simulink model "AOCS_FDIR"  (R2020b)
settings: Solver=ode45  StartTime=0.0  StopTime=200  FixedStep=1e-4  MaxStep=0.25  RelTol=1e-8  AbsTol=1e-8
values from neighbouring files (symbols this model uses):
  Gyros = zeros(3,6)    [Generate_Data.m]
  ReWhe = zeros(3,4)    [Generate_Data.m]
  Thrus = ones(1,8)    [Generate_Data.m]
undefined symbols (not defined in the file or in its folder): A, A_FEEP, A_FEEP_real, A_mag, CG_real, d_face, Dipole_SC, e0_0, e1_0, e2_0, e3_0, e_max_att, e_max_orb, Env_Drag, Env_J2, Env_Moon, Env_Sun, Env_TGG, Env_TMag, FEEP, g, GNSS, gyr, h_ref, h_RW, h_rw_0, I, I_real, IAU, initial_date_JD, J2, K_det, k_quat, km, m, mag, mu, mu_Moon, mu_Sun, n, n_orbits, q_0, Re, RW1, RW2, RW3, RW4, rx0, ry0, rz0, s, sigma1, sigma2, star, T_friction, th_2_gyr, th_FR_gyr, th_RW, th_SD_gyr_null, th_thruster ... (+10)
libraries: dspstat3 x16, aerolibutil x8, sharedutil x6, sharedtransform x5, vrlib x3, aerolibtransform2 x3, aerolibcelestial x2, aerolibobsolete x1, dspinverses x1
(part 2 of 4)

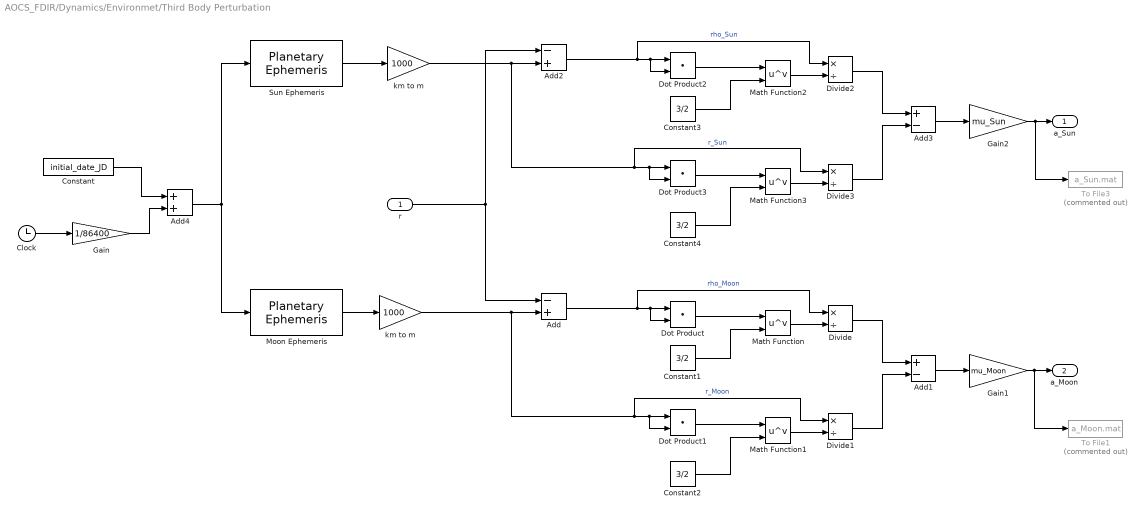
== system AOCS_FDIR/Dynamics/Environmet/Third Body Perturbation ==
  r : Inport
  Add : Sum  Inputs=-+
  Add1 : Sum  Inputs=+-
  Add2 : Sum  Inputs=-+
  Add3 : Sum  Inputs=+-
  Add4 : Sum
  Clock : Clock
  Constant : Constant  Value=initial_date_JD
  Constant{1..4} (4 alike) : Constant  Value=3/2
  Divide{,1..3} (4 alike) : Product  Inputs=*/
  Dot Product{,1..3} (4 alike) : DotProduct  InputSameDT=on  OutDataTypeStr=Inherit: Inherit via internal rule
  Gain : Gain  Gain=1/86400
  Gain1 : Gain  Gain=mu_Moon
  Gain2 : Gain  Gain=mu_Sun
  Math Function{,1..3} (4 alike) : Math  Operator=pow  SignedPower=on  SaturateOnIntegerOverflow=on
  Moon Ephemeris : aerolibcelestial/Planetary Ephemeris  kmflag=km,km/s  epochflag=Julian date  de=DE432t  nCenter=Earth  nTarget=Moon  errorflag=Warning  velflag=off
      settings: SourceProductBaseCode=AE
  Sun Ephemeris : aerolibcelestial/Planetary Ephemeris  kmflag=km,km/s  epochflag=Julian date  de=DE432t  nCenter=Earth  nTarget=Sun  errorflag=Warning  velflag=off
      settings: SourceProductBaseCode=AE
  To File1 : ToFile  Commented=on  Filename=a_Moon.mat  MatrixName=a_Moon
  To File3 : ToFile  Commented=on  Filename=a_Sun.mat  MatrixName=a_Sun
  "km to m " : Gain  Gain=1000
  "km to m " : Gain  Gain=1000
  a_Sun : Outport  VectorParamsAs1DForOutWhenUnconnected=off
  a_Moon : Outport  Port=2  VectorParamsAs1DForOutWhenUnconnected=off
  wires:
  Clock/1 -> Gain/1
  Moon Ephemeris/1 -> "km to m "/1
  r/1 -> Add/1, Add2/1
  Add/1 -> Divide/1, Dot Product/2, Dot Product/1  "rho_Moon"
  Dot Product/1 -> Math Function/1
  Constant1/1 -> Math Function/2
  Math Function/1 -> Divide/2
  Dot Product1/1 -> Math Function1/1
  Constant2/1 -> Math Function1/2
  Math Function1/1 -> Divide1/2
  Divide/1 -> Add1/1
  Divide1/1 -> Add1/2
  Add1/1 -> Gain1/1
  Gain1/1 -> To File1/1, a_Moon/1
  Divide2/1 -> Add3/1
  Math Function3/1 -> Divide3/2
  Constant4/1 -> Math Function3/2
  Dot Product3/1 -> Math Function3/1
  Math Function2/1 -> Divide2/2
  Add3/1 -> Gain2/1
  Add2/1 -> Divide2/1, Dot Product2/2, Dot Product2/1  "rho_Sun"
  Divide3/1 -> Add3/2
  Gain2/1 -> To File3/1, a_Sun/1
  Sun Ephemeris/1 -> "km to m "/1
  Dot Product2/1 -> Math Function2/1
  Constant3/1 -> Math Function2/2
  "km to m "/1 -> Divide1/1, Dot Product1/1, Dot Product1/2, Add/2  "r_Moon"
  "km to m "/1 -> Divide3/1, Dot Product3/1, Dot Product3/2, Add2/2  "r_Sun"
  Constant/1 -> Add4/1
  Gain/1 -> Add4/2
  Add4/1 -> Moon Ephemeris/1, Sun Ephemeris/1

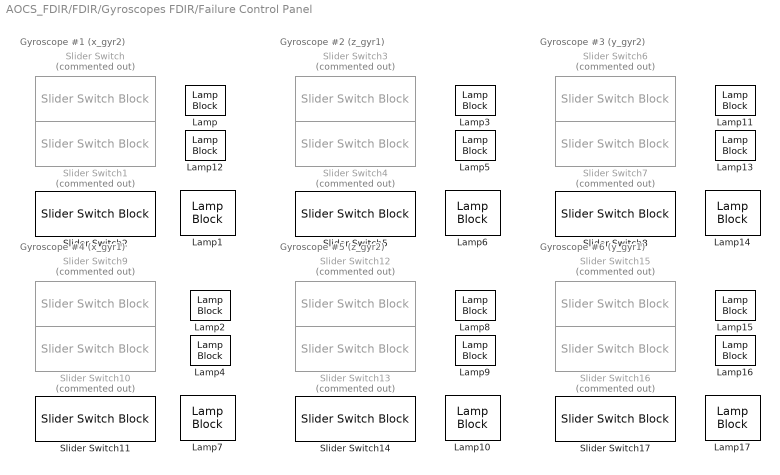
== system AOCS_FDIR/FDIR/Gyroscopes FDIR/Failure Control Panel ==
  note: Gyroscope #1 (x_gyr2)
  note: Gyroscope #2 (z_gyr1)
  note: Gyroscope #3 (y_gyr2)
  note: Gyroscope #4 (x_gyr1)
  note: Gyroscope #5 (z_gyr2)
  note: Gyroscope #6 (y_gyr1)
  Lamp{,1..17} (18 alike) : LampBlock  LabelPosition=Hide
  Slider Switch{,1,3..4,6..7,9..10,12..13,15..16} (12 alike) : SliderSwitchBlock  Commented=on
      settings: Values={{'Off', 'On'}, [0 1]}
  Slider Switch{2,5,8,11,14,17} (6 alike) : SliderSwitchBlock
      settings: Values={{'Off', 'On'}, [0 1]}

== system AOCS_FDIR/FDIR/Gyroscopes FDIR/Level 1 ==
  Diagnosis Frozen Signal : Subsystem
  Diagnosis Sudden Death : Subsystem
  MATLAB Function : MATLAB Function  TreatAsAtomicUnit=on
  Memory : Memory  InitialCondition=zeros(6,1)  InheritSampleTime=on
  Signal Specification : SignalSpecification  Dimensions=[6 1]
  tag scope: flagLevel1=global
  wires:
  MATLAB Function/1(flagLevel1) -> Signal Specification/1
  Diagnosis Sudden Death/1(flag_SD) -> MATLAB Function/1(flag_SD)
  Diagnosis Frozen Signal/1(flag_FR) -> MATLAB Function/2(flag_FR)
  Signal Specification/1 -> Memory/1
  Memory/1 -> [flagLevel1]

== system AOCS_FDIR/FDIR/Gyroscopes FDIR/Level 2 ==
  Clock : Clock
  Constant : Constant  Value=th_2_gyr
  Constant1 : Constant  Value=gyr.rate
  Constant2 : Constant  Value=win_length
  Constant3 : Constant  Value=win_length
  Constant4 : Constant  Value=sigma1
  Constant5 : Constant  Value=sigma2
  Evaluation : MATLAB Function  TreatAsAtomicUnit=on  SystemSampleTime=gyr.rate
  Fault Detection : MATLAB Function  TreatAsAtomicUnit=on
  GLR Test : MATLAB Function  TreatAsAtomicUnit=on
  Memory : Memory  InitialCondition=zeros(6,1)  InheritSampleTime=on
  Mux : Mux  Inputs=6
  Residuals Generator : MATLAB Function  TreatAsAtomicUnit=on  SystemSampleTime=gyr.rate
  Scope : Scope  NumInputPorts=9
  Scope1 : Scope  NumInputPorts=10
  Signal Specification : SignalSpecification  Dimensions=[6 1]
  tag scope: flagLevel2=global
  wires:
  [w_gyr] -> Residuals Generator/1(w_gyr)
  Mux/1 -> Signal Specification/1
  Fault Detection/1(flagm1) -> Mux/1
  Fault Detection/2(flagm2) -> Mux/2
  Fault Detection/3(flagm3) -> Mux/3
  Fault Detection/4(flagm4) -> Mux/4
  Fault Detection/5(flagm5) -> Mux/5
  Fault Detection/6(flagm6) -> Mux/6
  Signal Specification/1 -> Memory/1
  Memory/1 -> [flagLevel2]
  Residuals Generator/1(r1) -> GLR Test/1(r1)
  Residuals Generator/2(r2) -> GLR Test/2(r2)
  Residuals Generator/3(r3) -> GLR Test/3(r3)
  Residuals Generator/4(r4) -> GLR Test/4(r4)
  Residuals Generator/5(r5) -> GLR Test/5(r5)
  Residuals Generator/6(r6) -> GLR Test/6(r6)
  Residuals Generator/7(r7) -> GLR Test/7(r7)
  Residuals Generator/8(r8) -> GLR Test/8(r8)
  Residuals Generator/9(r9) -> GLR Test/9(r9)
  Constant3/1 -> GLR Test/10(win_length)
  Constant4/1 -> GLR Test/11(sigma1)
  Constant5/1 -> GLR Test/12(sigma2)
  Clock/1 -> GLR Test/13(t)
  Constant1/1 -> GLR Test/14(gyr_rate)
  GLR Test/1(S1) -> Scope/1, Evaluation/1(S1)
  GLR Test/2(S2) -> Scope/2, Evaluation/2(S2)
  GLR Test/3(S3) -> Scope/3, Evaluation/3(S3)
  GLR Test/4(S4) -> Scope/4, Evaluation/4(S4)
  GLR Test/5(S5) -> Scope/5, Evaluation/5(S5)
  GLR Test/6(S6) -> Scope/6, Evaluation/6(S6)
  GLR Test/7(S7) -> Scope/7, Evaluation/7(S7)
  GLR Test/8(S8) -> Scope/8, Evaluation/8(S8)
  GLR Test/9(S9) -> Scope/9, Evaluation/9(S9)
  Constant2/1 -> Evaluation/10(win_length)
  Constant/1 -> Evaluation/11(th)
  Evaluation/10(flag) -> Scope1/10, Fault Detection/10(flag)
  Evaluation/9(flagr9) -> Scope1/9, Fault Detection/9(flagr9)
  Evaluation/8(flagr8) -> Scope1/8, Fault Detection/8(flagr8)
  Evaluation/7(flagr7) -> Scope1/7, Fault Detection/7(flagr7)
  Evaluation/6(flagr6) -> Scope1/6, Fault Detection/6(flagr6)
  Evaluation/5(flagr5) -> Scope1/5, Fault Detection/5(flagr5)
  Evaluation/4(flagr4) -> Scope1/4, Fault Detection/4(flagr4)
  Evaluation/3(flagr3) -> Scope1/3, Fault Detection/3(flagr3)
  Evaluation/2(flagr2) -> Scope1/2, Fault Detection/2(flagr2)
  Evaluation/1(flagr1) -> Scope1/1, Fault Detection/1(flagr1)

== system AOCS_FDIR/FDIR/Reaction Wheels FDIR/Failure Control Panel ==
  note: Artificial Failure. RW #1
  note: Artificial Failure. RW #2
  note: Artificial Failure. RW #3
  note: Artificial Failure. RW #4
  Lamp{1..3,5} (4 alike) : LampBlock  LabelPosition=Hide
  Slider Switch{1..12} (12 alike) : SliderSwitchBlock  Commented=on
      settings: Values={{'Off', 'On'}, [0 1]}

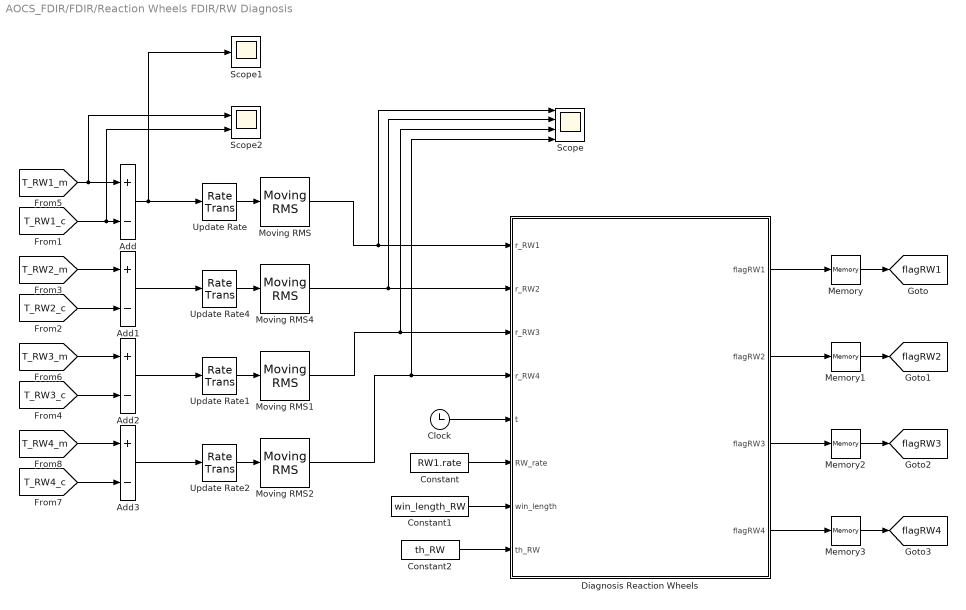
== system AOCS_FDIR/FDIR/Reaction Wheels FDIR/RW Diagnosis ==
  Add{,1..3} (4 alike) : Sum  Inputs=+-
  Clock : Clock
  Constant : Constant  Value=RW1.rate
  Constant1 : Constant  Value=win_length_RW
  Constant2 : Constant  Value=th_RW
  Diagnosis Reaction Wheels : MATLAB Function  TreatAsAtomicUnit=on
  Memory{,1..3} (4 alike) : Memory
  Moving RMS{,1..2,4} (4 alike) : dspstat3/Moving RMS  Method=Sliding window  ForgettingFactorPort=off  SpecifyWindowLength=on  WindowLength=win_length_RW  ForgettingFactor=0.9  SimulateUsing=Code generation
      settings: SourceProductBaseCode=DS
  Scope : Scope  NumInputPorts=4
  Scope1 : Scope
  Scope2 : Scope  NumInputPorts=2
  Update Rate : RateTransition  OutPortSampleTime=RW1.rate
  Update Rate1 : RateTransition  OutPortSampleTime=RW3.rate
  Update Rate2 : RateTransition  OutPortSampleTime=RW4.rate
  Update Rate4 : RateTransition  OutPortSampleTime=RW2.rate
  tag scope: flagRW1=global, flagRW2=global, flagRW3=global, flagRW4=global
  wires:
  Diagnosis Reaction Wheels/1(flagRW1) -> Memory/1
  Diagnosis Reaction Wheels/2(flagRW2) -> Memory1/1
  Diagnosis Reaction Wheels/3(flagRW3) -> Memory2/1
  Diagnosis Reaction Wheels/4(flagRW4) -> Memory3/1
  [T_RW1_m] -> Add/1, Scope2/1
  [T_RW1_c] -> Scope2/2, Add/2
  [T_RW2_m] -> Add1/1
  [T_RW2_c] -> Add1/2
  [T_RW3_m] -> Add2/1
  [T_RW3_c] -> Add2/2
  [T_RW4_m] -> Add3/1
  [T_RW4_c] -> Add3/2
  Add/1 -> Scope1/1, Update Rate/1
  Add1/1 -> Update Rate4/1
  Add2/1 -> Update Rate1/1
  Add3/1 -> Update Rate2/1
  Memory/1 -> [flagRW1]
  Memory1/1 -> [flagRW2]
  Memory2/1 -> [flagRW3]
  Memory3/1 -> [flagRW4]
  Moving RMS/1 -> Scope/1, Diagnosis Reaction Wheels/1(r_RW1)
  Update Rate/1 -> Moving RMS/1
  Moving RMS4/1 -> Scope/2, Diagnosis Reaction Wheels/2(r_RW2)
  Update Rate4/1 -> Moving RMS4/1
  Moving RMS1/1 -> Diagnosis Reaction Wheels/3(r_RW3), Scope/3
  Update Rate1/1 -> Moving RMS1/1
  Moving RMS2/1 -> Scope/4, Diagnosis Reaction Wheels/4(r_RW4)
  Update Rate2/1 -> Moving RMS2/1
  Clock/1 -> Diagnosis Reaction Wheels/5(t)
  Constant/1 -> Diagnosis Reaction Wheels/6(RW_rate)
  Constant1/1 -> Diagnosis Reaction Wheels/7(win_length)
  Constant2/1 -> Diagnosis Reaction Wheels/8(th_RW)

== system AOCS_FDIR/FDIR/Thrusters FDIR/Failure Control Panel ==
  Lamp{,1..7} (8 alike) : LampBlock  LabelPosition=Hide
  Slider Switch{,1..7} (8 alike) : SliderSwitchBlock  Commented=on
      settings: Values={{'Off', 'On'}, [1 0]}

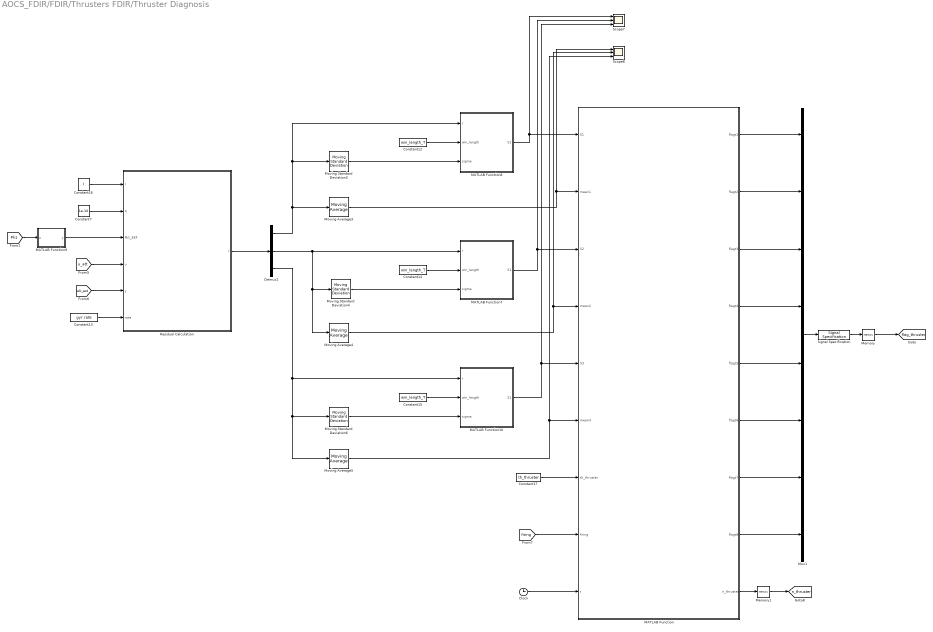
== system AOCS_FDIR/FDIR/Thrusters FDIR/Thruster Diagnosis ==
  Clock : Clock
  Constant12 : Constant  Value=win_length_T
  Constant13 : Constant  Value=gyr.rate
  Constant14 : Constant  Value=win_length_T
  Constant15 : Constant  Value=win_length_T
  Constant16 : Constant  Value=I
  Constant17 : Constant  Value=th_thruster
  Constant7 : Constant  Value=1e-10
  Demux2 : Demux  Outputs=3
  MATLAB Function : MATLAB Function  TreatAsAtomicUnit=on
  MATLAB Function10 : MATLAB Function  TreatAsAtomicUnit=on  SystemSampleTime=gyr.rate
  MATLAB Function7 : MATLAB Function  TreatAsAtomicUnit=on  SystemSampleTime=gyr.rate
  MATLAB Function8 : MATLAB Function  TreatAsAtomicUnit=on  SystemSampleTime=gyr.rate
  MATLAB Function9 : MATLAB Function  TreatAsAtomicUnit=on
  Memory : Memory  InitialCondition=zeros(8,1)  InheritSampleTime=on
  Memory1 : Memory  InitialCondition=8  InheritSampleTime=on
  Moving Average3 : dspstat3/Moving Average  Method=Sliding window  ForgettingFactorPort=off  SpecifyWindowLength=on  WindowLength=win_length_T  ForgettingFactor=0.9  SimulateUsing=Code generation
  Moving Average4 : dspstat3/Moving Average  Method=Sliding window  ForgettingFactorPort=off  SpecifyWindowLength=on  WindowLength=win_length_T  ForgettingFactor=0.9  SimulateUsing=Code generation
  Moving Average5 : dspstat3/Moving Average  Method=Sliding window  ForgettingFactorPort=off  SpecifyWindowLength=on  WindowLength=win_length_T  ForgettingFactor=0.9  SimulateUsing=Code generation
  Moving Standard Deviation3 : dspstat3/Moving Standard Deviation  Method=Sliding window  ForgettingFactorPort=off  SpecifyWindowLength=on  WindowLength=win_length_T  ForgettingFactor=0.9  SimulateUsing=Code generation
      settings: SourceProductBaseCode=DS
  Moving Standard Deviation4 : dspstat3/Moving Standard Deviation  Method=Sliding window  ForgettingFactorPort=off  SpecifyWindowLength=on  WindowLength=win_length_T  ForgettingFactor=0.9  SimulateUsing=Code generation
      settings: SourceProductBaseCode=DS
  Moving Standard Deviation6 : dspstat3/Moving Standard Deviation  Method=Sliding window  ForgettingFactorPort=off  SpecifyWindowLength=on  WindowLength=win_length_T  ForgettingFactor=0.9  SimulateUsing=Code generation
      settings: SourceProductBaseCode=DS
  Mux1 : Mux  Inputs=8
  Residual Calculation : MATLAB Function  TreatAsAtomicUnit=on  SystemSampleTime=gyr.rate
  Scope7 : Scope  NumInputPorts=3
  Scope8 : Scope  NumInputPorts=3
  Signal Specification : SignalSpecification  Dimensions=[8 1]
  tag scope: flag_thruster=global, n_thruster=global
  wires:
  [Pk1] -> MATLAB Function9/1(u)
  [u_att] -> Residual Calculation/4(u)
  [wb_est] -> Residual Calculation/5(y)
  Constant7/1 -> Residual Calculation/2(q)
  Constant16/1 -> Residual Calculation/1(I)
  MATLAB Function9/1(y) -> Residual Calculation/3(Pk1_EKF)
  Residual Calculation/1(r) -> Demux2/1
  Demux2/1 -> Moving Average3/1, MATLAB Function8/1(r), Moving Standard Deviation3/1
  Moving Standard Deviation3/1 -> MATLAB Function8/3(sigma)
  Constant12/1 -> MATLAB Function8/2(win_length)
  Constant13/1 -> Residual Calculation/6(rate)
  Demux2/2 -> Moving Average4/1, Moving Standard Deviation4/1, MATLAB Function7/1(r)
  Moving Standard Deviation4/1 -> MATLAB Function7/3(sigma)
  Constant14/1 -> MATLAB Function7/2(win_length)
  Constant15/1 -> MATLAB Function10/2(win_length)
  Moving Standard Deviation6/1 -> MATLAB Function10/3(sigma)
  Demux2/3 -> MATLAB Function10/1(r), Moving Average5/1, Moving Standard Deviation6/1
  MATLAB Function8/1(S1) -> Scope7/1, MATLAB Function/1(S1)
  MATLAB Function7/1(S1) -> Scope7/2, MATLAB Function/3(S2)
  MATLAB Function10/1(S1) -> Scope7/3, MATLAB Function/5(S3)
  Moving Average3/1 -> Scope8/1, MATLAB Function/2(mean1)
  Moving Average4/1 -> Scope8/2, MATLAB Function/4(mean2)
  Moving Average5/1 -> Scope8/3, MATLAB Function/6(mean3)
  Constant17/1 -> MATLAB Function/7(th_thruster)
  [firing] -> MATLAB Function/8(firing)
  MATLAB Function/1(flagt1) -> Mux1/1
  MATLAB Function/2(flagt2) -> Mux1/2
  MATLAB Function/3(flagt3) -> Mux1/3
  MATLAB Function/4(flagt4) -> Mux1/4
  MATLAB Function/5(flagt5) -> Mux1/5
  MATLAB Function/7(flagt7) -> Mux1/7
  MATLAB Function/6(flagt6) -> Mux1/6
  MATLAB Function/8(flagt8) -> Mux1/8
  MATLAB Function/9(n_thruster) -> Memory1/1
  Mux1/1 -> Signal Specification/1
  Memory/1 -> [flag_thruster]
  Signal Specification/1 -> Memory/1
  Memory1/1 -> [n_thruster]
  Clock/1 -> MATLAB Function/9(t)

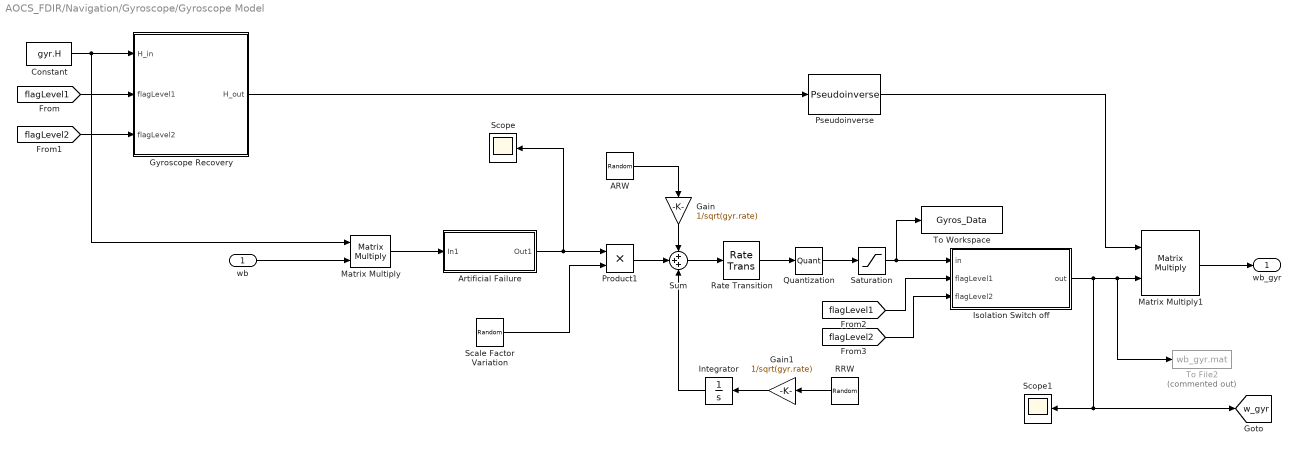
== system AOCS_FDIR/Navigation/Gyroscope/Gyroscope Model ==
  wb : Inport
  ARW : RandomNumber  Variance=(gyr.ARW)^2  Seed=[7; 8; 9;10;11;12]
  Artificial Failure : Subsystem
  Constant : Constant  Value=gyr.H
  Gain : Gain  Gain=1/sqrt(gyr.rate)
  Gain1 : Gain  Gain=1/sqrt(gyr.rate)
  Gyroscope Recovery : MATLAB Function  TreatAsAtomicUnit=on
  Integrator : Integrator  InitialCondition=gyr.bias*ones(6,1)
  "Isolation Switch off " : MATLAB Function  TreatAsAtomicUnit=on
  Matrix Multiply : Product  Multiplication=Matrix(*)
  Matrix Multiply1 : Product  Multiplication=Matrix(*)
  Product1 : Product
  Pseudoinverse : dspinverses/Pseudoinverse  wanterr=off  SimulateUsing=Interpreted execution
      settings: SourceProductBaseCode=DS
  Quantization : Quantizer  QuantizationInterval=2*gyr.range/(2^gyr.bits-1)
  RRW : RandomNumber  Variance=(gyr.RRW)^2  Seed=[21;22;23;24;25;26]
  Rate Transition : RateTransition  InitialCondition=gyr.H*w_SC_0  OutPortSampleTime=gyr.rate
  Saturation : Saturate  UpperLimit=gyr.range*ones(6,1)  LowerLimit=-gyr.range*ones(6,1)
  Scale Factor Variation : UniformRandomNumber  Minimum=(100-gyr.scale)/100  Maximum=(100+gyr.scale)/100  Seed=[67;68;69;70;71;72]
  Scope : Scope
  Scope1 : Scope
  Sum : Sum  Inputs=+++
  To File2 : ToFile  Commented=on  Filename=wb_gyr.mat  MatrixName=wb_gyr
  To Workspace : ToWorkspace  VariableName=Gyros_Data  SaveFormat=Timeseries  SampleTime=-1
  wb_gyr : Outport  VectorParamsAs1DForOutWhenUnconnected=off
  tag scope: w_gyr=global
  wires:
  RRW/1 -> Gain1/1
  Gain1/1 -> Integrator/1
  Gain/1 -> Sum/1
  Integrator/1 -> Sum/3
  ARW/1 -> Gain/1
  wb/1 -> Matrix Multiply/2
  Scale Factor Variation/1 -> Product1/2
  Product1/1 -> Sum/2
  Sum/1 -> Rate Transition/1
  Rate Transition/1 -> Quantization/1
  Quantization/1 -> Saturation/1
  Constant/1 -> Matrix Multiply/1, Gyroscope Recovery/1(H_in)
  [flagLevel1] -> Gyroscope Recovery/2(flagLevel1)
  [flagLevel2] -> Gyroscope Recovery/3(flagLevel2)
  Gyroscope Recovery/1(H_out) -> Pseudoinverse/1
  Matrix Multiply/1 -> Artificial Failure/1(In1)
  Pseudoinverse/1 -> Matrix Multiply1/1
  Matrix Multiply1/1 -> wb_gyr/1
  Artificial Failure/1(Out1) -> Scope/1, Product1/1
  [flagLevel1] -> "Isolation Switch off "/2(flagLevel1)
  [flagLevel2] -> "Isolation Switch off "/3(flagLevel2)
  Saturation/1 -> To Workspace/1, "Isolation Switch off "/1(in)
  "Isolation Switch off "/1(out) -> Scope1/1, [w_gyr], To File2/1, Matrix Multiply1/2

== system AOCS_FDIR/Control/Attitude Control/Reaction Wheel Model/Artificial Failure1 ==
  In1 : Inport
  In2 : Inport  Port=2
  Accuracy Loss : Constant  Value=ReWhe(3,1)
  Clock : Clock
  Constant : Constant  Value=T_friction
  Constant1 : Constant  Value=0  VectorParams1D=off
  Friction Failure : Constant  Value=ReWhe(2,1)
  MATLAB Function : MATLAB Function  TreatAsAtomicUnit=on
  Motor Failure : Constant  Value=ReWhe(1,1)
  Switch : Switch  Criteria=u2 > Threshold  Threshold=25+(150*rand)
  Switch1 : Switch  Criteria=u2 > Threshold  Threshold=25+(150*rand)
  Switch2 : Switch  Criteria=u2 > Threshold  Threshold=25+(150*rand)
  Out1 : Outport  VectorParamsAs1DForOutWhenUnconnected=off
  wires:
  In1/1 -> MATLAB Function/1(in)
  MATLAB Function/1(out) -> Out1/1
  In2/1 -> MATLAB Function/2(h_RW)
  Constant/1 -> MATLAB Function/3(T_friction)
  Clock/1 -> Switch2/2, Switch1/2, Switch/2
  Switch/1 -> MATLAB Function/4(flag1)
  Switch2/1 -> MATLAB Function/6(flag3)
  Switch1/1 -> MATLAB Function/5(flag2)
  Accuracy Loss/1 -> Switch2/3
  Friction Failure/1 -> Switch1/3
  Motor Failure/1 -> Switch/3
  Constant1/1 -> Switch/1, Switch1/1, Switch2/1

== system AOCS_FDIR/Control/Attitude Control/Reaction Wheel Model/Artificial Failure2 ==
  In1 : Inport
  In2 : Inport  Port=2
  Accuracy Loss : Constant  Value=ReWhe(3,2)
  Clock : Clock
  Constant : Constant  Value=T_friction
  Constant1 : Constant  Value=0  VectorParams1D=off
  Friction Failure : Constant  Value=ReWhe(2,2)
  MATLAB Function : MATLAB Function  TreatAsAtomicUnit=on
  Motor Failure : Constant  Value=ReWhe(1,2)
  Switch : Switch  Criteria=u2 > Threshold  Threshold=25+(150*rand)
  Switch1 : Switch  Criteria=u2 > Threshold  Threshold=25+(150*rand)
  Switch2 : Switch  Criteria=u2 > Threshold  Threshold=25+(150*rand)
  Out1 : Outport  VectorParamsAs1DForOutWhenUnconnected=off
  wires:
  In1/1 -> MATLAB Function/1(in)
  MATLAB Function/1(out) -> Out1/1
  In2/1 -> MATLAB Function/2(h_RW)
  Constant/1 -> MATLAB Function/3(T_friction)
  Constant1/1 -> Switch/1, Switch1/1, Switch2/1
  Friction Failure/1 -> Switch1/3
  Motor Failure/1 -> Switch/3
  Clock/1 -> Switch2/2, Switch1/2, Switch/2
  Accuracy Loss/1 -> Switch2/3
  Switch/1 -> MATLAB Function/4(flag1)
  Switch1/1 -> MATLAB Function/5(flag2)
  Switch2/1 -> MATLAB Function/6(flag3)

== system AOCS_FDIR/Control/Attitude Control/Reaction Wheel Model/Artificial Failure3 ==
  In1 : Inport
  In2 : Inport  Port=2
  Accuracy Loss : Constant  Value=ReWhe(3,3)
  Clock : Clock
  Constant : Constant  Value=T_friction
  Constant1 : Constant  Value=0  VectorParams1D=off
  Friction Failure : Constant  Value=ReWhe(2,3)
  MATLAB Function : MATLAB Function  TreatAsAtomicUnit=on
  Motor Failure : Constant  Value=ReWhe(1,3)
  Switch : Switch  Criteria=u2 > Threshold  Threshold=25+(150*rand)
  Switch1 : Switch  Criteria=u2 > Threshold  Threshold=25+(150*rand)
  Switch2 : Switch  Criteria=u2 > Threshold  Threshold=25+(150*rand)
  Out1 : Outport  VectorParamsAs1DForOutWhenUnconnected=off
  wires:
  In1/1 -> MATLAB Function/1(in)
  MATLAB Function/1(out) -> Out1/1
  In2/1 -> MATLAB Function/2(h_RW)
  Constant/1 -> MATLAB Function/3(T_friction)
  Constant1/1 -> Switch/1, Switch1/1, Switch2/1
  Friction Failure/1 -> Switch1/3
  Motor Failure/1 -> Switch/3
  Clock/1 -> Switch2/2, Switch1/2, Switch/2
  Accuracy Loss/1 -> Switch2/3
  Switch/1 -> MATLAB Function/4(flag1)
  Switch1/1 -> MATLAB Function/5(flag2)
  Switch2/1 -> MATLAB Function/6(flag3)

== system AOCS_FDIR/Control/Attitude Control/Reaction Wheel Model/Artificial Failure4 ==
  In1 : Inport
  In2 : Inport  Port=2
  Accuracy Loss : Constant  Value=ReWhe(3,4)
  Clock : Clock
  Constant : Constant  Value=T_friction
  Constant1 : Constant  Value=0  VectorParams1D=off
  Friction Failure : Constant  Value=ReWhe(2,4)
  MATLAB Function : MATLAB Function  TreatAsAtomicUnit=on
  Motor Failure : Constant  Value=ReWhe(1,4)
  Switch : Switch  Criteria=u2 > Threshold  Threshold=25+(150*rand)
  Switch1 : Switch  Criteria=u2 > Threshold  Threshold=25+(150*rand)
  Switch2 : Switch  Criteria=u2 > Threshold  Threshold=25+(150*rand)
  Out1 : Outport  VectorParamsAs1DForOutWhenUnconnected=off
  wires:
  In1/1 -> MATLAB Function/1(in)
  MATLAB Function/1(out) -> Out1/1
  In2/1 -> MATLAB Function/2(h_RW)
  Constant/1 -> MATLAB Function/3(T_friction)
  Constant1/1 -> Switch/1, Switch1/1, Switch2/1
  Friction Failure/1 -> Switch1/3
  Motor Failure/1 -> Switch/3
  Clock/1 -> Switch2/2, Switch1/2, Switch/2
  Accuracy Loss/1 -> Switch2/3
  Switch/1 -> MATLAB Function/4(flag1)
  Switch1/1 -> MATLAB Function/5(flag2)
  Switch2/1 -> MATLAB Function/6(flag3)

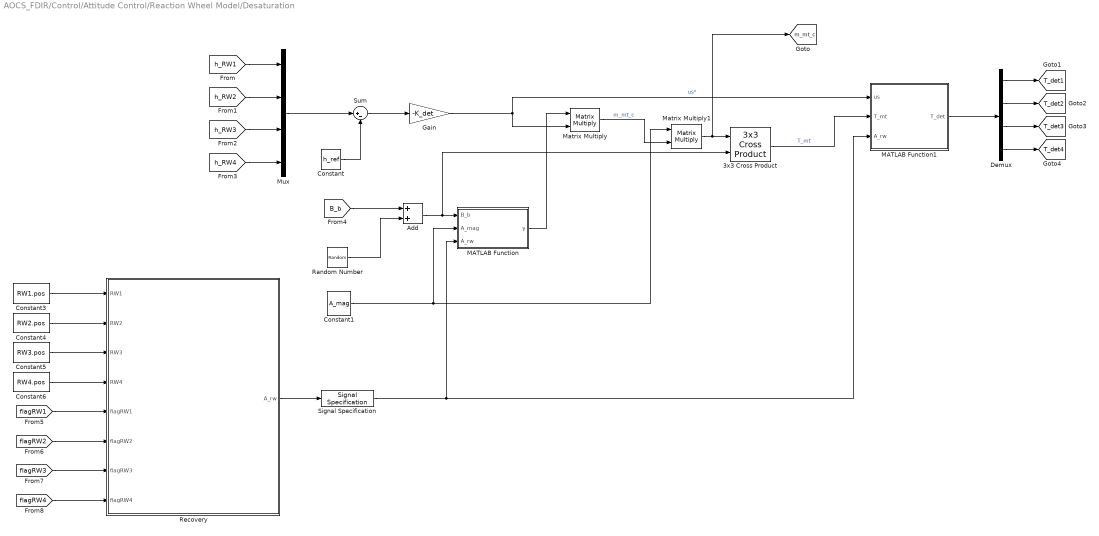
== system AOCS_FDIR/Control/Attitude Control/Reaction Wheel Model/Desaturation ==
  3x3 Cross Product : sharedutil/3x3 Cross Product  aMode=aMode
      settings: SourceProductBaseCode=AE,PW,MT,UV,VE,VP
  Add : Sum
  Constant : Constant  Value=h_ref
  Constant1 : Constant  Value=A_mag
  Constant3 : Constant  Value=RW1.pos
  Constant4 : Constant  Value=RW2.pos
  Constant5 : Constant  Value=RW3.pos
  Constant6 : Constant  Value=RW4.pos
  Demux : Demux
  Gain : Gain  Gain=-K_det
  MATLAB Function : MATLAB Function  TreatAsAtomicUnit=on
  MATLAB Function1 : MATLAB Function  TreatAsAtomicUnit=on
  Matrix Multiply : Product  Multiplication=Matrix(*)
  Matrix Multiply1 : Product  Multiplication=Matrix(*)
  Mux : Mux
  Random Number : RandomNumber  Variance=mag.noise^2  Seed=[23441 23442 23443]  SampleTime=mag.rate
  Recovery : MATLAB Function  TreatAsAtomicUnit=on
  Signal Specification : SignalSpecification  Dimensions=[3 4]
  Sum : Sum  Inputs=|+-
  tag scope: T_det1=global, T_det2=global, T_det3=global, T_det4=global, m_mt_c=global
  wires:
  [h_RW1] -> Mux/1
  [h_RW2] -> Mux/2
  [h_RW3] -> Mux/3
  [h_RW4] -> Mux/4
  Mux/1 -> Sum/1
  Constant/1 -> Sum/2
  Sum/1 -> Gain/1
  Gain/1 -> MATLAB Function1/1(us), Matrix Multiply/2  "us*"
  Random Number/1 -> Add/2
  [B_b] -> Add/1
  Add/1 -> 3x3 Cross Product/2, MATLAB Function/1(B_b)
  Constant1/1 -> MATLAB Function/2(A_mag), Matrix Multiply1/1
  Recovery/1(A_rw) -> Signal Specification/1
  MATLAB Function/1(y) -> Matrix Multiply/1
  Matrix Multiply/1 -> Matrix Multiply1/2  "m_mt_c"
  Matrix Multiply1/1 -> [m_mt_c], 3x3 Cross Product/1
  3x3 Cross Product/1 -> MATLAB Function1/2(T_mt)  "T_mt"
  MATLAB Function1/1(T_det) -> Demux/1
  Demux/1 -> [T_det1]
  Demux/2 -> [T_det2]
  Demux/3 -> [T_det3]
  Demux/4 -> [T_det4]
  [flagRW1] -> Recovery/5(flagRW1)
  Constant6/1 -> Recovery/4(RW4)
  [flagRW2] -> Recovery/6(flagRW2)
  Constant3/1 -> Recovery/1(RW1)
  Constant4/1 -> Recovery/2(RW2)
  [flagRW4] -> Recovery/8(flagRW4)
  [flagRW3] -> Recovery/7(flagRW3)
  Constant5/1 -> Recovery/3(RW3)
  Signal Specification/1 -> MATLAB Function/3(A_rw), MATLAB Function1/3(A_rw)

== system AOCS_FDIR/Control/Attitude Control/Reaction Wheel Model/Isolation1 ==
  In1 : Inport
  In2 : Inport  Port=2
  Constant : Constant  Value=T_friction
  Hit Crossing : HitCross
  MATLAB Function : MATLAB Function  TreatAsAtomicUnit=on
  Out1 : Outport  VectorParamsAs1DForOutWhenUnconnected=off
  wires:
  In1/1 -> MATLAB Function/1(T_in)
  MATLAB Function/1(T_out) -> Out1/1
  In2/1 -> MATLAB Function/3(h_RW), Hit Crossing/1
  Hit Crossing/1 -> MATLAB Function/2(stop)
  [flagRW1] -> MATLAB Function/5(flagRW)
  Constant/1 -> MATLAB Function/4(T_friction)

== system AOCS_FDIR/Control/Attitude Control/Reaction Wheel Model/Isolation2 ==
  In1 : Inport
  In2 : Inport  Port=2
  Constant : Constant  Value=T_friction
  Hit Crossing : HitCross
  MATLAB Function : MATLAB Function  TreatAsAtomicUnit=on
  Out1 : Outport  VectorParamsAs1DForOutWhenUnconnected=off
  wires:
  In1/1 -> MATLAB Function/1(T_in)
  MATLAB Function/1(T_out) -> Out1/1
  In2/1 -> MATLAB Function/3(h_RW), Hit Crossing/1
  Hit Crossing/1 -> MATLAB Function/2(stop)
  [flagRW2] -> MATLAB Function/5(flagRW)
  Constant/1 -> MATLAB Function/4(T_friction)

== system AOCS_FDIR/Control/Attitude Control/Reaction Wheel Model/Isolation3 ==
  In1 : Inport
  In2 : Inport  Port=2
  Constant : Constant  Value=T_friction
  Hit Crossing : HitCross
  MATLAB Function : MATLAB Function  TreatAsAtomicUnit=on
  Out1 : Outport  VectorParamsAs1DForOutWhenUnconnected=off
  wires:
  In1/1 -> MATLAB Function/1(T_in)
  MATLAB Function/1(T_out) -> Out1/1
  In2/1 -> MATLAB Function/3(h_RW), Hit Crossing/1
  Hit Crossing/1 -> MATLAB Function/2(stop)
  [flagRW3] -> MATLAB Function/5(flagRW)
  Constant/1 -> MATLAB Function/4(T_friction)

== system AOCS_FDIR/Control/Attitude Control/Reaction Wheel Model/Isolation4 ==
  In1 : Inport
  In2 : Inport  Port=2
  Constant : Constant  Value=T_friction
  Hit Crossing : HitCross
  MATLAB Function : MATLAB Function  TreatAsAtomicUnit=on
  Out1 : Outport  VectorParamsAs1DForOutWhenUnconnected=off
  wires:
  In1/1 -> MATLAB Function/1(T_in)
  MATLAB Function/1(T_out) -> Out1/1
  In2/1 -> MATLAB Function/3(h_RW), Hit Crossing/1
  Hit Crossing/1 -> MATLAB Function/2(stop)
  [flagRW4] -> MATLAB Function/5(flagRW)
  Constant/1 -> MATLAB Function/4(T_friction)

== system AOCS_FDIR/Control/Orbit Control/Thruster Model/Artificial Failure ==
  In1 : Inport
  Clock : Clock
  Constant : Constant  Value=Thrus
  Constant1 : Constant  Value=ones(1,8)
  Demux : Demux  Outputs=8
  MATLAB Function : MATLAB Function  TreatAsAtomicUnit=on
  Switch : Switch  Criteria=u2 > Threshold  Threshold=25+(150*rand)
  Out1 : Outport  VectorParamsAs1DForOutWhenUnconnected=off
  wires:
  In1/1 -> MATLAB Function/1(in)
  MATLAB Function/1(out) -> Out1/1
  Demux/1 -> MATLAB Function/2(flag1)
  Demux/8 -> MATLAB Function/9(flag8)
  Demux/7 -> MATLAB Function/8(flag7)
  Demux/6 -> MATLAB Function/7(flag6)
  Demux/4 -> MATLAB Function/5(flag4)
  Demux/5 -> MATLAB Function/6(flag5)
  Demux/3 -> MATLAB Function/4(flag3)
  Demux/2 -> MATLAB Function/3(flag2)
  Switch/1 -> Demux/1
  Constant/1 -> Switch/3
  Constant1/1 -> Switch/1
  Clock/1 -> Switch/2

== system AOCS_FDIR/Dynamics/6DOF Model/Attitude Kinematics/Quaternion Evolution ==
  p q r : Inport
  q0 q1 q2 q3 : Inport  Port=2
  Constant : Constant
  Dot Product : DotProduct  OutDataTypeStr=Inherit: Inherit via internal rule
  High Gain Quaternion Normalization : Gain  Gain=k_quat  SaturateOnIntegerOverflow=on  OutDataTypeStr=Inherit: Same as input  ParamDataTypeStr=Inherit: Same as input
  Mux1 : Mux  Inputs=[3 4 1]
  Mux2 : Mux
  Sum : Sum  Inputs=|+-  InputSameDT=on  SaturateOnIntegerOverflow=on  OutDataTypeStr=Inherit: Same as first input
  q0dot : Fcn  Expr=-0.5 * ( u[5]*u[1]+u[6]*u[2]+u[7]*u[3] ) + u[8]*u[4]
  q1dot : Fcn  Expr=0.5 * ( u[4]*u[1]+u[6]*u[3]-u[7]*u[2] ) + u[8]*u[5]
  q2dot : Fcn  Expr=0.5 * ( u[4]*u[2]+u[7]*u[1]-u[5]*u[3] ) + u[8]*u[6]
  q3dot : Fcn  Expr=0.5 * ( u[4]*u[3]+u[5]*u[2]-u[6]*u[1] ) + u[8]*u[7]
  qdot : Outport  InitialOutput=0  VectorParamsAs1DForOutWhenUnconnected=off
  wires:
  Dot Product/1 -> Sum/2
  High Gain Quaternion Normalization/1 -> Mux1/3
  p q r/1 -> Mux1/1
  q0 q1 q2 q3/1 -> Mux1/2, Dot Product/2, Dot Product/1
  Sum/1 -> High Gain Quaternion Normalization/1
  q0dot/1 -> Mux2/1
  Mux2/1 -> qdot/1
  q1dot/1 -> Mux2/2
  Mux1/1 -> q1dot/1, q0dot/1, q3dot/1, q2dot/1
  q3dot/1 -> Mux2/4
  q2dot/1 -> Mux2/3
  Constant/1 -> Sum/1

== system AOCS_FDIR/FDIR/Gyroscopes FDIR/Level 1/Diagnosis Frozen Signal ==
  Clock1 : Clock
  Constant4 : Constant  Value=th_FR_gyr
  Constant5 : Constant  Value=win_length
  Constant6 : Constant  Value=gyr.rate
  Demux1 : Demux  Outputs=6
  MATLAB Function : MATLAB Function  TreatAsAtomicUnit=on
  Moving Standard Deviation{3..8} (6 alike) : dspstat3/Moving Standard Deviation  Method=Sliding window  ForgettingFactorPort=off  SpecifyWindowLength=on  WindowLength=win_length  ForgettingFactor=0.9  SimulateUsing=Code generation
      settings: SourceProductBaseCode=DS
  Mux : Mux  Inputs=6
  Rate Transition6 : RateTransition  OutPortSampleTime=gyr.rate
  Scope : Scope
  Signal Specification : SignalSpecification  Dimensions=[6 1]
  To File2 : ToFile  Commented=on  Filename=FS.mat  MatrixName=FS
  flag_FR : Outport  VectorParamsAs1DForOutWhenUnconnected=off
  wires:
  [w_gyr] -> Rate Transition6/1
  Moving Standard Deviation3/1 -> To File2/1, Scope/1, MATLAB Function/1(std_1)
  Moving Standard Deviation4/1 -> MATLAB Function/2(std_2)
  Moving Standard Deviation5/1 -> MATLAB Function/3(std_3)
  Moving Standard Deviation6/1 -> MATLAB Function/4(std_4)
  Moving Standard Deviation7/1 -> MATLAB Function/5(std_5)
  Moving Standard Deviation8/1 -> MATLAB Function/6(std_6)
  Constant4/1 -> MATLAB Function/7(th_FR_gyr)
  Constant5/1 -> MATLAB Function/8(win_length)
  Constant6/1 -> MATLAB Function/9(gyr_rate)
  Clock1/1 -> MATLAB Function/10(t)
  MATLAB Function/1(flag_FR_1) -> Mux/1
  MATLAB Function/5(flag_FR_5) -> Mux/5
  Mux/1 -> Signal Specification/1
  MATLAB Function/3(flag_FR_3) -> Mux/3
  MATLAB Function/2(flag_FR_2) -> Mux/2
  MATLAB Function/4(flag_FR_4) -> Mux/4
  MATLAB Function/6(flag_FR_6) -> Mux/6
  Signal Specification/1 -> flag_FR/1
  Demux1/1 -> Moving Standard Deviation3/1
  Demux1/2 -> Moving Standard Deviation4/1
  Demux1/3 -> Moving Standard Deviation5/1
  Demux1/4 -> Moving Standard Deviation6/1
  Demux1/5 -> Moving Standard Deviation7/1
  Demux1/6 -> Moving Standard Deviation8/1
  Rate Transition6/1 -> Demux1/1

== system AOCS_FDIR/FDIR/Gyroscopes FDIR/Level 1/Diagnosis Sudden Death ==
  Abs{3..8} (6 alike) : Abs
  Constant4 : Constant  Value=th_SD_gyr_null
  Demux1 : Demux  Outputs=6
  Derivative{3..8} (6 alike) : Derivative
  Diagnosis Sudden Death Gyroscope : MATLAB Function  TreatAsAtomicUnit=on
  Hit Crossing{3..8} (6 alike) : HitCross  HitCrossingOffset=th_SD_gyr_der
  Mux : Mux  Inputs=6
  Scope : Scope  NumInputPorts=6
  Scope1 : Scope  NumInputPorts=6
  Signal Specification : SignalSpecification  Dimensions=[6 1]
  flag_SD : Outport  VectorParamsAs1DForOutWhenUnconnected=off
  wires:
  Demux1/1 -> Diagnosis Sudden Death Gyroscope/2(m1), Derivative3/1
  Derivative3/1 -> Abs3/1
  Abs3/1 -> Scope/1, Hit Crossing3/1
  Abs4/1 -> Scope/2, Hit Crossing4/1
  Demux1/2 -> Diagnosis Sudden Death Gyroscope/4(m2), Derivative4/1
  Derivative4/1 -> Abs4/1
  [w_gyr] -> Demux1/1
  Abs5/1 -> Scope/3, Hit Crossing5/1
  Demux1/3 -> Diagnosis Sudden Death Gyroscope/6(m3), Derivative5/1
  Derivative5/1 -> Abs5/1
  Abs6/1 -> Scope/4, Hit Crossing6/1
  Demux1/4 -> Diagnosis Sudden Death Gyroscope/8(m4), Derivative6/1
  Derivative6/1 -> Abs6/1
  Abs7/1 -> Scope/5, Hit Crossing7/1
  Demux1/5 -> Diagnosis Sudden Death Gyroscope/10(m5), Derivative7/1
  Derivative7/1 -> Abs7/1
  Abs8/1 -> Scope/6, Hit Crossing8/1
  Demux1/6 -> Diagnosis Sudden Death Gyroscope/12(m6), Derivative8/1
  Derivative8/1 -> Abs8/1
  Hit Crossing3/1 -> Diagnosis Sudden Death Gyroscope/1(dm1)
  Hit Crossing4/1 -> Diagnosis Sudden Death Gyroscope/3(dm2)
  Hit Crossing5/1 -> Diagnosis Sudden Death Gyroscope/5(dm3)
  Hit Crossing6/1 -> Diagnosis Sudden Death Gyroscope/7(dm4)
  Hit Crossing7/1 -> Diagnosis Sudden Death Gyroscope/9(dm5)
  Hit Crossing8/1 -> Diagnosis Sudden Death Gyroscope/11(dm6)
  Constant4/1 -> Diagnosis Sudden Death Gyroscope/13(th_SD_gyr_null)
  Diagnosis Sudden Death Gyroscope/1(flag_SD_1) -> Scope1/1, Mux/1
  Diagnosis Sudden Death Gyroscope/2(flag_SD_2) -> Scope1/2, Mux/2
  Diagnosis Sudden Death Gyroscope/3(flag_SD_3) -> Scope1/3, Mux/3
  Diagnosis Sudden Death Gyroscope/4(flag_SD_4) -> Scope1/4, Mux/4
  Diagnosis Sudden Death Gyroscope/5(flag_SD_5) -> Scope1/5, Mux/5
  Diagnosis Sudden Death Gyroscope/6(flag_SD_6) -> Scope1/6, Mux/6
  Mux/1 -> Signal Specification/1
  Signal Specification/1 -> flag_SD/1

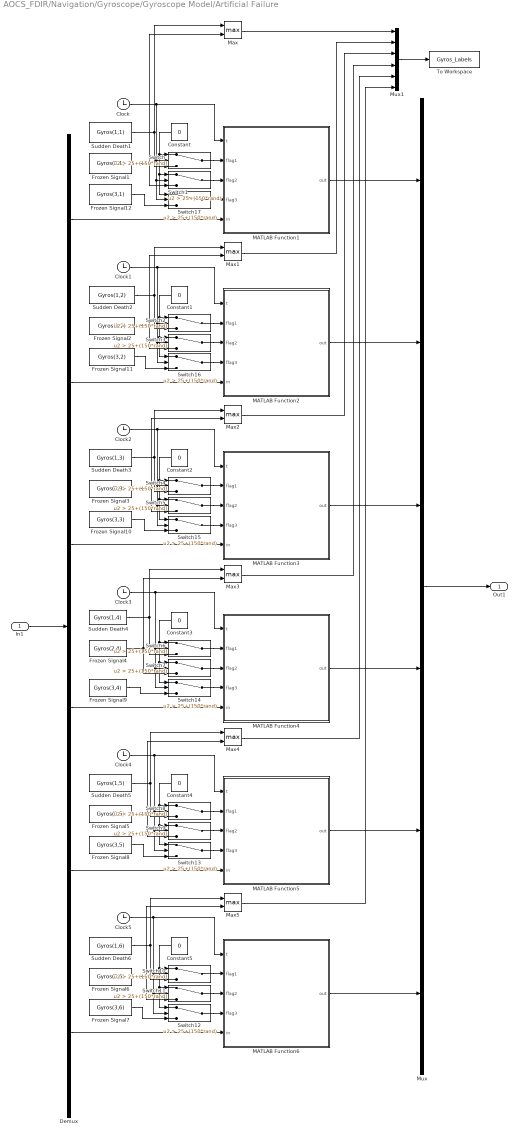
== system AOCS_FDIR/Navigation/Gyroscope/Gyroscope Model/Artificial Failure ==
  In1 : Inport
  Clock{,1..5} (6 alike) : Clock
  Constant{,1..5} (6 alike) : Constant  Value=0
  Demux : Demux  Outputs=6
  Frozen Signal1 : Constant  Value=Gyros(2,1)
  Frozen Signal10 : Constant  Value=Gyros(3,3)
  Frozen Signal11 : Constant  Value=Gyros(3,2)
  Frozen Signal12 : Constant  Value=Gyros(3,1)
  Frozen Signal2 : Constant  Value=Gyros(2,2)
  Frozen Signal3 : Constant  Value=Gyros(2,3)
  Frozen Signal4 : Constant  Value=Gyros(2,4)
  Frozen Signal5 : Constant  Value=Gyros(2,5)
  Frozen Signal6 : Constant  Value=Gyros(2,6)
  Frozen Signal7 : Constant  Value=Gyros(3,6)
  Frozen Signal8 : Constant  Value=Gyros(3,5)
  Frozen Signal9 : Constant  Value=Gyros(3,4)
  MATLAB Function1 : MATLAB Function  TreatAsAtomicUnit=on
  MATLAB Function2 : MATLAB Function  TreatAsAtomicUnit=on
  MATLAB Function3 : MATLAB Function  TreatAsAtomicUnit=on
  MATLAB Function4 : MATLAB Function  TreatAsAtomicUnit=on
  MATLAB Function5 : MATLAB Function  TreatAsAtomicUnit=on
  MATLAB Function6 : MATLAB Function  TreatAsAtomicUnit=on
  Max{,1..5} (6 alike) : MinMax  Function=max  Inputs=2
  Mux : Mux  Inputs=6
  Mux1 : Mux  Inputs=6
  Sudden Death1 : Constant  Value=Gyros(1,1)
  Sudden Death2 : Constant  Value=Gyros(1,2)
  Sudden Death3 : Constant  Value=Gyros(1,3)
  Sudden Death4 : Constant  Value=Gyros(1,4)
  Sudden Death5 : Constant  Value=Gyros(1,5)
  Sudden Death6 : Constant  Value=Gyros(1,6)
  Switch{,1..17} (18 alike) : Switch  Criteria=u2 > Threshold  Threshold=25+(150*rand)
  To Workspace : ToWorkspace  VariableName=Gyros_Labels  SampleTime=-1
      settings: MaxDataPoints=1
  Out1 : Outport  VectorParamsAs1DForOutWhenUnconnected=off
  wires:
  In1/1 -> Demux/1
  Demux/1 -> MATLAB Function1/5(in)
  Clock/1 -> MATLAB Function1/1(t), Switch/2, Switch17/2, Switch1/2
  Clock1/1 -> Switch16/2, Switch3/2, Switch2/2, MATLAB Function2/1(t)
  Demux/2 -> MATLAB Function2/5(in)
  Clock2/1 -> Switch15/2, Switch5/2, Switch4/2, MATLAB Function3/1(t)
  Demux/3 -> MATLAB Function3/5(in)
  Clock3/1 -> Switch6/2, Switch14/2, Switch7/2, MATLAB Function4/1(t)
  Demux/4 -> MATLAB Function4/5(in)
  Clock4/1 -> Switch13/2, Switch9/2, Switch8/2, MATLAB Function5/1(t)
  Demux/5 -> MATLAB Function5/5(in)
  Clock5/1 -> Switch12/2, Switch11/2, Switch10/2, MATLAB Function6/1(t)
  Demux/6 -> MATLAB Function6/5(in)
  MATLAB Function1/1(out) -> Mux/1
  MATLAB Function2/1(out) -> Mux/2
  MATLAB Function3/1(out) -> Mux/3
  MATLAB Function4/1(out) -> Mux/4
  MATLAB Function5/1(out) -> Mux/5
  MATLAB Function6/1(out) -> Mux/6
  Mux/1 -> Out1/1
  Switch/1 -> MATLAB Function1/2(flag1)
  Switch1/1 -> MATLAB Function1/3(flag2)
  Constant/1 -> Switch17/1, Switch1/1, Switch/1
  Switch2/1 -> MATLAB Function2/2(flag1)
  Switch3/1 -> MATLAB Function2/3(flag2)
  Constant1/1 -> Switch16/1, Switch3/1, Switch2/1
  Switch4/1 -> MATLAB Function3/2(flag1)
  Switch5/1 -> MATLAB Function3/3(flag2)
  Constant2/1 -> Switch15/1, Switch5/1, Switch4/1
  Switch6/1 -> MATLAB Function4/2(flag1)
  Switch7/1 -> MATLAB Function4/3(flag2)
  Constant3/1 -> Switch14/1, Switch7/1, Switch6/1
  Switch8/1 -> MATLAB Function5/2(flag1)
  Switch9/1 -> MATLAB Function5/3(flag2)
  Constant4/1 -> Switch13/1, Switch9/1, Switch8/1
  Frozen Signal5/1 -> Max4/2, Switch9/3
  Sudden Death5/1 -> Max4/1, Switch8/3
  Switch10/1 -> MATLAB Function6/2(flag1)
  Switch11/1 -> MATLAB Function6/3(flag2)
  Constant5/1 -> Switch12/1, Switch11/1, Switch10/1
  Frozen Signal6/1 -> Max5/2, Switch11/3
  Sudden Death6/1 -> Max5/1, Switch10/3
  Mux1/1 -> To Workspace/1
  Max/1 -> Mux1/1
  Max1/1 -> Mux1/2
  Max2/1 -> Mux1/3
  Max3/1 -> Mux1/4
  Max4/1 -> Mux1/5
  Max5/1 -> Mux1/6
  Sudden Death1/1 -> Max/1, Switch/3
  Frozen Signal1/1 -> Max/2, Switch1/3
  Frozen Signal2/1 -> Max1/2, Switch3/3
  Sudden Death2/1 -> Max1/1, Switch2/3
  Frozen Signal3/1 -> Max2/2, Switch5/3
  Sudden Death3/1 -> Max2/1, Switch4/3
  Frozen Signal4/1 -> Switch7/3, Max3/2
  Sudden Death4/1 -> Switch6/3, Max3/1
  Switch12/1 -> MATLAB Function6/4(flag3)
  Frozen Signal7/1 -> Switch12/3
  Switch13/1 -> MATLAB Function5/4(flag3)
  Frozen Signal8/1 -> Switch13/3
  Switch14/1 -> MATLAB Function4/4(flag3)
  Frozen Signal9/1 -> Switch14/3
  Switch15/1 -> MATLAB Function3/4(flag3)
  Frozen Signal10/1 -> Switch15/3
  Switch16/1 -> MATLAB Function2/4(flag3)
  Frozen Signal11/1 -> Switch16/3
  Switch17/1 -> MATLAB Function1/4(flag3)
  Frozen Signal12/1 -> Switch17/3

== matlab function AOCS_FDIR/Guidance/MATLAB Function1 ==
  data: r input; DCM_Pointing_ECI output; v input
function DCM_Pointing_ECI = fcn(r,v)
%% Compute the rotation matrix to keep the body frame pointing to Nadir
i_Pointing = -r/norm(r);
k_Pointing = -cross(r,v)/norm(cross(r,v));
j_Pointing = -cross(i_Pointing,k_Pointing);

DCM_Pointing_ECI = [i_Pointing'; j_Pointing'; k_Pointing'];

== matlab function AOCS_FDIR/Control/Orbit Control/Atmospheric Density ==
  data: h input; rho output
function rho = Exponential_Atm_Model(h)
%% Initialization
rho = 0;

%% Parameters of the model
h_0   = [0; 25; 30; 35; 40; 45; 50; 55; 60; 65; 70; 75; 80; 85; 90; 95; 100; 110; 120; 130; 140; 150; 160; 180; 200; 250; 300; 350; 400; 450; 500; 600; 700; 800; 900; 1000];
rho_0 = [1.225; 3.899e-2; 1.774e-2; 8.279e-3; 3.972e-3; 1.995e-3; 1.057e-3; 5.821e-4; 3.206e-4; 1.718e-4; 8.770e-5; 4.178e-5; 1.905e-5; 8.337e-6; 3.396e-6; 1.343e-6; 5.297e-7; 9.661e-8; 2.438e-8; 8.484e-9; 3.845e-9; 2.070e-9; 1.224e-9; 5.464e-10; 2.789e-10; 7.248e-11; 2.418e-11; 9.158e-12; 3.725e-12; 1.585e-12; 6.967e-13; 1.454e-13; 3.614e-14; 1.170e-14; 5.245e-15; 3.019e-15];
H     = [8.44; 6.49; 6.75; 7.07; 7.47; 7.83; 7.95; 7.73; 7.29; 6.81; 6.33; 6.00; 5.70; 5.41; 5.38; 5.74; 6.15; 8.06; 11.6; 16.1; 20.6; 24.6; 26.3; 33.2; 38.5; 46.9; 52.5; 56.4; 59.4; 62.2; 65.8; 79; 109; 164; 225; 268];

%% Compute the density as a function of altitude
if h<=h_0(2)
    rho = rho_0(1)*exp(-(h-h_0(1))/H(1));
elseif h>h_0(end)
    rho = rho_0(end)*exp(-(h-h_0(end)/H(end)));
else
    for i=2:(length(h_0)-1)
        if h>h_0(i) && h<=h_0(i+1)
            rho = rho_0(i)*exp(-(h-h_0(i))/H(i));
        end
    end
end

end

== matlab function AOCS_FDIR/Control/Orbit Control/Thruster Allocation/MATLAB Function ==
  data: F input; F_thrusters output; A_FEEP input; firing output
% function [F, firing] = fcn(b_eq, A_eq, ub)
% coder.extrinsic('linprog')
% 
% c  = ones(8,1);
% lb = zeros(8,1);
% ub = ones(8,1)*ub;
% 
% sol1 = linprog(c,[],[],A_eq,b_eq,lb,ub);
% 
% if isempty(sol1)
%     sol2 = linprog(c,[],[],A_eq,[0;b_eq(2);0;0;0;0],lb,ub);
%     if isempty(sol2)
%         F =zeros(8,1);
%         firing = 0;
%     else
%         F = sol2;
%         firing = 1;
%     end
% else
%     F = sol1;
%     firing = 1;
% end

function [F_thrusters,firing]=fcn(F, A_FEEP)

F_thrusters = pinv(A_FEEP)*F;                                               % Distribute control effort between thrusters using pseudoiverse
ind = find(sign(F_thrusters)<0);                                            % Find thrusters with negative force (not possible!!)

if isempty(ind)
    firing = 1;
    return
else
    firing = 0;
    for i=1:length(ind)
        if F_thrusters(ind(i))>-1e-2                                        % Consider possible very small negative values due to computational errors
            F_thrusters(ind(i)) = 0;
            if i==length(ind)
                firing = 1;
                return
            end
        else
            F_thrusters = pinv(A_FEEP)*[0;F(2);0;0;0;0];                    % Try to only counteract the drag if there is no solution for multiple correction
            firing = 0;
        end
    end
end


ind = find(sign(F_thrusters)<0);

if isempty(ind)
    firing = 1;
    return
else
    firing = 0;
    for i=1:length(ind)
        if F_thrusters(ind(i))>-1e-2                                        % Consider possible very small negative values due to computational errors
            F_thrusters(ind(i)) = 0;
            if i==length(ind)
                firing = 1;
                return
            end
        else
            F_thrusters = zeros(8,1);                                       % There is no solution
            firing = 0;
        end
    end
end

end

== matlab function AOCS_FDIR/Control/Orbit Control/Orbit Controller/MATLAB Function ==
  data: R input; a output; V input; e output; i output; RA output; w output; u output
function [a, e, i, RA, w, u] = sv2coe(R,V)
%-------------------------------------------------------------------------
% This function computes the classical orbital elements (coe)
% from the state vector (R,V).
%
% mu - gravitational parameter (mˆ3/sˆ2)
% R - position vector in ECI (m)
% V - velocity vector in ECI (m)
% r, v - the moduli of R and V
% vr - radial velocity component (m/s)
% H - the angular momentum vector (mˆ2/s)
% h - the moduli of H (mˆ2/s)
% i - inclination of the orbit (rad)
% N - the node line vector (mˆ2/s)
% n - the moduli of N
% cp - cross product of N and R
% RA - right ascension of the ascending node (rad)
% E - eccentricity vector
% e - eccentricity (moduli of E)
% eps - a small number below which the eccentricity is
% considered to be zero
% w - argument of perigee (rad)
% TA - true anomaly (rad)
% a - semimajor axis (m)
% coe - vector of orbital elements [a, e, i, RA, w, TA]
%
% ------------------------------------------------------------------------
%% Inputs
mu = 3.986004418e14;
eps = 1.e-10;

r = norm(R);
v = norm(V);
vr = dot(R,V)/r;

H = cross(R,V);
h = norm(H);

%% Inclination
i = acos(H(3)/h);

%% Node line
N = cross([0 0 1],H);
n = norm(N);

%% Right Ascension
if n ~= 0
    RA = acos(N(1)/n);
    if N(2) < 0
        RA = 2*pi - RA;
    end
else
    RA= 0;                 % No defined asceding node (Equatorial orbit)
end

%% Eccentricity
E = 1/mu*((v^2 - mu/r)*R - r*vr*V);
e = norm(E);

%% Argument of periapsis
% To avoid numerical errors
d_N_E=dot(N,E)/n/e;
if d_N_E>1 
    d_N_E = 1;
elseif d_N_E<-1
    d_N_E = -1;
end

if n ~= 0
    if e > eps
        w = acos(d_N_E);
        if E(3) < 0
            w = 2*pi - w;
        end
    else
        w = 0;             % No defined periapsis (Circular orbit)    
    end
else
    w = 0;                 % No defined ascending node (Equatorial orbits)
end


%% True anomaly
% To avoid numerical errors
d_E_R=dot(E,R)/e/r;
if d_E_R>1 
    d_E_R = 1;
elseif d_E_R<-1
    d_E_R = -1;
end

d_N_R=dot(N,R)/n/r;
if d_N_R>1 
    d_N_R = 1;
elseif d_N_R<-1
    d_N_R = -1;
end

if e > eps
    TA = norm(acos(d_E_R));
    if vr < 0
        TA = 2*pi - TA;
    end
else
    cp = cross(N,R);
    if cp(3) >= 0
        TA = acos(d_N_R);
    else
        TA = 2*pi - acos(d_N_R);
    end
end

%% Semimajor axis
a = h^2/mu/(1 - e^2);

%% Mean latitude
M = 2*atan(sqrt((1-e)/(1+e))*tan(TA/2))-...
    (e*sqrt(1-e^2)*sin(TA))/(1+e*cos(TA));
u = w + M;

== matlab function AOCS_FDIR/Control/Orbit Control/Orbit Controller/MATLAB Function1 ==
  data: R input; a output; V input; e output; i output; RA output; w output; u output
function [a, e, i, RA, w, u] = sv2coe(R,V)
%-------------------------------------------------------------------------
% This function computes the classical orbital elements (coe)
% from the state vector (R,V).
%
% mu - gravitational parameter (mˆ3/sˆ2)
% R - position vector in ECI (m)
% V - velocity vector in ECI (m)
% r, v - the moduli of R and V
% vr - radial velocity component (m/s)
% H - the angular momentum vector (mˆ2/s)
% h - the moduli of H (mˆ2/s)
% i - inclination of the orbit (rad)
% N - the node line vector (mˆ2/s)
% n - the moduli of N
% cp - cross product of N and R
% RA - right ascension of the ascending node (rad)
% E - eccentricity vector
% e - eccentricity (moduli of E)
% eps - a small number below which the eccentricity is
% considered to be zero
% w - argument of perigee (rad)
% TA - true anomaly (rad)
% a - semimajor axis (m)
% coe - vector of orbital elements [a, e, i, RA, w, TA]
%
% ------------------------------------------------------------------------
%% Inputs
mu = 3.986004418e14;
eps = 1.e-10;

r = norm(R);
v = norm(V);
vr = dot(R,V)/r;

H = cross(R,V);
h = norm(H);

%% Inclination
i = acos(H(3)/h);

%% Node line
N = cross([0 0 1],H);
n = norm(N);

%% Right Ascension
if n ~= 0
    RA = acos(N(1)/n);
    if N(2) < 0
        RA = 2*pi - RA;
    end
else
    RA= 0;                 % No defined asceding node (Equatorial orbit)
end

%% Eccentricity
E = 1/mu*((v^2 - mu/r)*R - r*vr*V);
e = norm(E);

%% Argument of periapsis
% To avoid numerical errors
d_N_E=dot(N,E)/n/e;
if d_N_E>1 
    d_N_E = 1;
elseif d_N_E<-1
    d_N_E = -1;
end

if n ~= 0
    if e > eps
        w = acos(d_N_E);
        if E(3) < 0
            w = 2*pi - w;
        end
    else
        w = 0;             % No defined periapsis (Circular orbit)    
    end
else
    w = 0;                 % No defined ascending node (Equatorial orbits)
end


%% True anomaly
% To avoid numerical errors
d_E_R=dot(E,R)/e/r;
if d_E_R>1 
    d_E_R = 1;
elseif d_E_R<-1
    d_E_R = -1;
end

d_N_R=dot(N,R)/n/r;
if d_N_R>1 
    d_N_R = 1;
elseif d_N_R<-1
    d_N_R = -1;
end

if e > eps
    TA = norm(acos(d_E_R));
    if vr < 0
        TA = 2*pi - TA;
    end
else
    cp = cross(N,R);
    if cp(3) >= 0
        TA = acos(d_N_R);
    else
        TA = 2*pi - acos(d_N_R);
    end
end

%% Semimajor axis
a = h^2/mu/(1 - e^2);

%% Mean latitude
M = 2*atan(sqrt((1-e)/(1+e))*tan(TA/2))-...
    (e*sqrt(1-e^2)*sin(TA))/(1+e*cos(TA));
u = w + M;
